simulink library "INT_FlFWLvl_DD"  (R2016b)
settings: Solver=VariableStepAuto  StartTime=0.0  StopTime=10.0  RelTol=1e-3
settings Model: Creator=liutao  LastModifiedBy=liutao

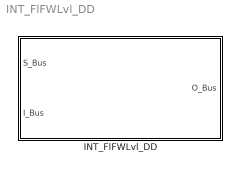
== system INT_FlFWLvl_DD ==
  INT_FlFWLvl_DD : Subsystem

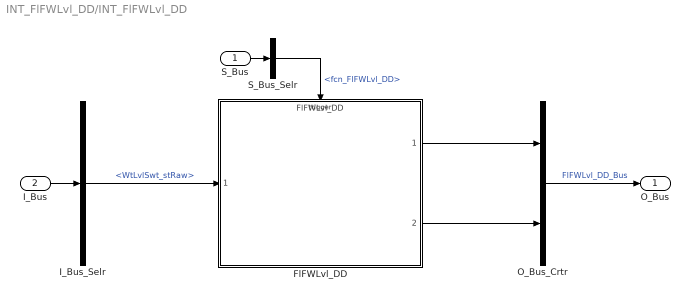
== system INT_FlFWLvl_DD/INT_FlFWLvl_DD ==
  S_Bus : Inport
  I_Bus : Inport  Port=2
  FlFWLvl_DD : ModelReference  ModelNameDialog=FlFWLvl_DD  SimulationMode=Normal  ModelReferenceVersion=1.14  TriggerPortName=function  TriggerPortTriggerType=function-call  TriggerPortStatesWhenEnabling=held
  I_Bus_Selr : BusSelector  OutputSignals=WtLvlSwt_stRaw
  O_Bus_Crtr : BusCreator  Inputs=2
  S_Bus_Selr : BusSelector  OutputSignals=fcn_FlFWLvl_DD
  O_Bus : Outport
  wires:
  S_Bus_Selr/1 -> FlFWLvl_DD/Trigger  "<fcn_FlFWLvl_DD>"
  S_Bus/1 -> S_Bus_Selr/1
  I_Bus/1 -> I_Bus_Selr/1
  I_Bus_Selr/1 -> FlFWLvl_DD/1  "<WtLvlSwt_stRaw>"
  O_Bus_Crtr/1 -> O_Bus/1  "FlFWLvl_DD_Bus"
  FlFWLvl_DD/1 -> O_Bus_Crtr/1
  FlFWLvl_DD/2 -> O_Bus_Crtr/2
